simulink model "ZS042"  (R2016b)
settings: Solver=FixedStepAuto  StartTime=0.0  StopTime=inf  RelTol=1e-3  EnableMultiTasking=on
PreLoadFcn:
  | addpath(genpath('../../Drivers'))
libraries: arduinoDrivers_lib x2
settings Model: SimulationMode=external  ExtModeTrigDuration=2  Creator=Raphael  LastModifiedBy=Raphael
settings OptimizationCC: MaxStackSize=64
settings DebuggingCC: ParameterTunabilityLossMsg=error
settings HardwareCC: ProdBitPerInt=16  ProdBitPerPointer=16  ProdBitPerSizeT=16  ProdBitPerPtrDiffT=16  ProdLargestAtomicFloat=None  ProdWordSize=8  ProdHWDeviceType=Atmel->AVR
settings RTWCC: SystemTargetFile=ert.tlc  HardwareBoard=Arduino Mega 2560  TLCOptions=-aInlineSetEventsForThisBaseRateFcn=TLC_FALSE -aSuppressMultiTaskScheduler=TLC_FALSE -aRateBasedStepFcn=1  TemplateMakefile=ert_default_tmf  Description=Embedded Coder  GenerateReport=on  Toolchain=Arduino AVR v1.6.7  BuildConfiguration=Faster Runs  IncludeHyperlinkInReport=on  GenerateTraceInfo=on  GenerateTraceReport=on  GenerateTraceReportSl=on  GenerateTraceReportSf=on  GenerateTraceReportEml=on
settings CodeAppCC: ForceParamTrailComments=on  IgnoreCustomStorageClasses=off  OperatorAnnotations=on  SimulinkDataObjDesc=on  SFDataObjDesc=on  MATLABFcnDesc=on  InsertBlockDesc=on  MATLABSourceComments=on
settings ERTTargetCC: SupportContinuousTime=on  SupportVariableSizeSignals=on

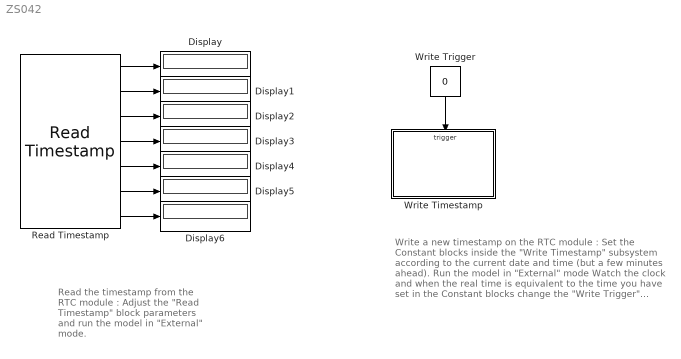
== system ZS042 ==
  note: Write a new timestamp on the RTC module :
      |
      | Set the Constant blocks inside the "Write Timestamp" subsystem according to the current date and time (but a few minutes ahead).
      | Run the model in "External" mode
      | Watch the clock and when the real time is equivalent to the time you have set in the Constant blocks change the "Write Trigger" Constant block value from 0 to 1 suddenly.
  note: Read the timestamp from the RTC module :
      |
      | Adjust the "Read Timestamp" block parameters and run the model in "External" mode.
  Display{,1..6} (7 alike) : Display
  Read Timestamp : arduinoDrivers_lib/ZS042 Real-Time-Clock/Read Timestamp  tsMask=1
  Write Timestamp : Subsystem
  Write Trigger : Constant  Value=0  OutDataTypeStr=uint8
  wires:
  Read Timestamp/1 -> Display/1
  Read Timestamp/2 -> Display1/1
  Read Timestamp/3 -> Display2/1
  Read Timestamp/4 -> Display3/1
  Read Timestamp/5 -> Display4/1
  Read Timestamp/6 -> Display5/1
  Read Timestamp/7 -> Display6/1
  Write Trigger/1 -> Write Timestamp/Trigger

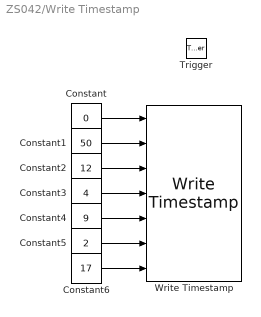
== system ZS042/Write Timestamp ==
  Trigger : TriggerPort  VariantControl=Variant  PortDimensions=1
  Constant : Constant  Value=0  OutDataTypeStr=uint8  SampleTime=-1
  Constant1 : Constant  Value=50  OutDataTypeStr=uint8  SampleTime=-1
  Constant2 : Constant  Value=12  OutDataTypeStr=uint8  SampleTime=-1
  Constant3 : Constant  Value=4  OutDataTypeStr=uint8  SampleTime=-1
  Constant4 : Constant  Value=9  OutDataTypeStr=uint8  SampleTime=-1
  Constant5 : Constant  Value=2  OutDataTypeStr=uint8  SampleTime=-1
  Constant6 : Constant  Value=17  OutDataTypeStr=uint8  SampleTime=-1
  Write Timestamp : arduinoDrivers_lib/ZS042 Real-Time-Clock/Write Timestamp
  wires:
  Constant1/1 -> Write Timestamp/2
  Constant/1 -> Write Timestamp/1
  Constant5/1 -> Write Timestamp/6
  Constant4/1 -> Write Timestamp/5
  Constant6/1 -> Write Timestamp/7
  Constant2/1 -> Write Timestamp/3
  Constant3/1 -> Write Timestamp/4
